simulink model "Modelo_NL_Ley_de_control_NL"  (R2017a)
settings: Solver=VariableStepAuto  StartTime=0.0  StopTime=2  MaxStep=1e-4  RelTol=1e-3
undefined symbols (not defined in the file): alfa_cu, beq, Cts, Jeq, LambdaM, Ld, Lq, Pp, Rs, Rsref, Rts_amb, Tamb, Tleq, Tsref
settings Model: Creator=merem  LastModifiedBy=merem

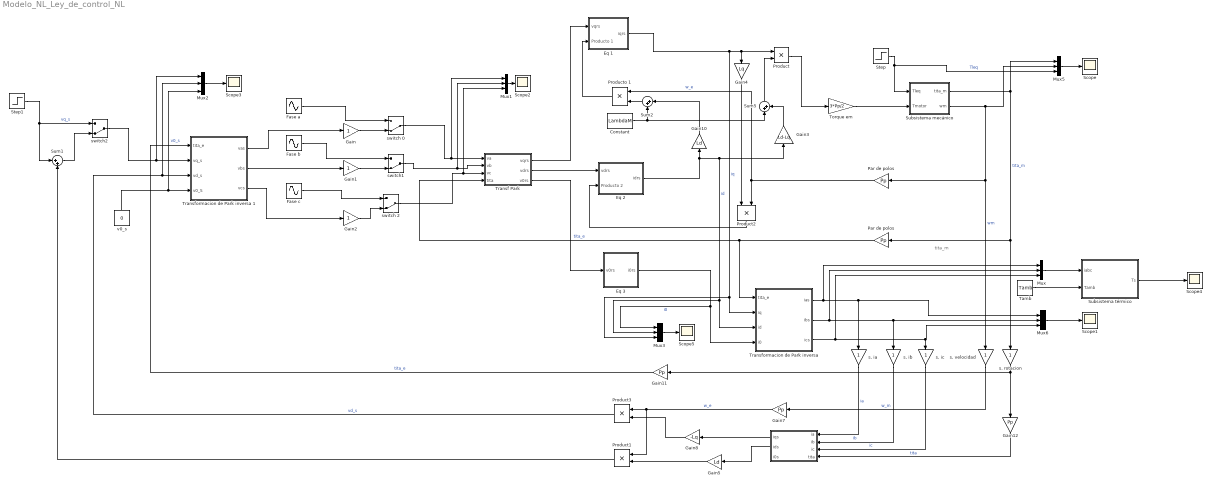
== system Modelo_NL_Ley_de_control_NL ==
  note: tita_m
  " " : Subsystem
  Constant : Constant  Value=LambdaM
  Eq 1 : Subsystem
  "Eq 2 " : Subsystem
  Eq 3 : Subsystem
  Fase a : Sin  SampleTime=0
  Fase b : Sin  SampleTime=0
  Fase c : Sin  SampleTime=0
  Gain : Gain
  Gain1 : Gain
  Gain10 : Gain  Gain=Ld
  Gain11 : Gain  Gain=Pp
  Gain12 : Gain  Gain=Pp
  Gain2 : Gain
  Gain3 : Gain  Gain=Ld-Lq
  Gain4 : Gain  Gain=Lq
  Gain5 : Gain  Gain=Ld
  Gain7 : Gain  Gain=Pp
  Gain8 : Gain  Gain=-Lq
  Mux{,1..3,5..6} (6 alike) : Mux  Inputs=3
  Par de polos : Gain  Gain=Pp
  "Par de polos " : Gain  Gain=Pp
  Product{,1..3} (4 alike) : Product
  Producto 1 : Product
  Scope{,1..5} (6 alike) : Scope
  Step : Step  Time=0  After=Tleq  SampleTime=0
  Step1 : Step  Time=0  After=20  SampleTime=0
  Subsistema mecánico : Subsystem
  Subsistema térmico : Subsystem
  Sum1 : Sum  Inputs=|++
  Sum2 : Sum  Inputs=|++
  Sum5 : Sum  Inputs=|++
  "Tamb " : Constant  Value=Tamb
  "Torque em " : Gain  Gain=3*Pp/2
  "Transf Park " : Subsystem
  "Transformacion de Park inversa " : Subsystem
  Transformacion de Park inversa 1 : Subsystem
  s. ia : Gain
  s. ib : Gain
  "s. ic " : Gain
  s. rotacion : Gain
  s. velocidad : Gain
  switch 0 : ManualSwitch  CurrentSetting=0
  "switch 2 " : ManualSwitch  CurrentSetting=0
  switch1 : ManualSwitch  CurrentSetting=0
  switch2 : ManualSwitch  CurrentSetting=0
  v0_s : Constant  Value=0
  wires:
  s. rotacion/1 -> Gain12/1, Gain11/1
  "s. ic "/1 -> " "/3("ic ")  "ic"
  "Transformacion de Park inversa "/1(ias) -> Mux/1, s. ia/1, Mux6/1
  Sum5/1 -> Product/2
  switch 0/1 -> Mux1/1, "Transf Park "/1("va ")
  Gain7/1 -> Product3/1, Product1/1  "w_e"
  Gain8/1 -> Product3/2
  switch1/1 -> Mux1/2, "Transf Park "/2(vb)
  s. ia/1 -> " "/1("ia ")  "ia"
  s. velocidad/1 -> Gain7/1  "w_m"
  "Torque em "/1 -> Subsistema mecánico/2("Tmotor ")
  Gain5/1 -> Product1/2
  "Eq 2 "/1("idrs ") -> Mux3/2, "Transformacion de Park inversa "/3(id), Gain3/1, Gain10/1  "id"
  Producto 1/1 -> Eq 1/2("Producto 1 ")
  Gain4/1 -> Product2/1
  Subsistema mecánico/1("tita_m ") -> "Par de polos "/1, s. rotacion/1, Mux5/1  "tita_m"
  Gain3/1 -> Sum5/2
  Step/1 -> Mux5/3, Subsistema mecánico/1("Tleq ")  "Tleq"
  Gain10/1 -> Sum2/1
  Eq 1/1("iqrs ") -> Mux3/3, "Transformacion de Park inversa "/2(iq), Gain4/1, Product/1  "iq"
  Gain1/1 -> switch1/2
  Gain2/1 -> "switch 2 "/2
  "switch 2 "/1 -> Mux1/3, "Transf Park "/3(vc)
  Fase c/1 -> "switch 2 "/1
  Product/1 -> "Torque em "/1
  Mux5/1 -> Scope/1
  Gain12/1 -> " "/4("tita ")  "tita"
  "Transformacion de Park inversa "/3("ics ") -> Mux/3, Mux6/3, "s. ic "/1
  v0_s/1 -> Mux2/3, Transformacion de Park inversa 1/4("v0_S ")  "v0_s"
  Product3/1 -> Mux2/2, Transformacion de Park inversa 1/3(vd_s)  "vd_s"
  s. ib/1 -> " "/2("ib ")  "ib"
  Fase b/1 -> switch1/1
  Par de polos/1 -> Producto 1/1, Product2/2  "w_e"
  Constant/1 -> Sum5/1, Sum2/2
  Mux6/1 -> Scope1/1
  Gain11/1 -> Transformacion de Park inversa 1/1(tita_e)  "tita_e"
  "Transf Park "/2("vdrs ") -> "Eq 2 "/1("vdrs ")
  Gain/1 -> switch 0/2
  Fase a/1 -> switch 0/1
  " "/2("ids ") -> Gain5/1
  "Transf Park "/1(vqrs) -> Eq 1/1(vqrs)
  "Par de polos "/1 -> "Transf Park "/4(tita), "Transformacion de Park inversa "/1(tita_e)  "tita_e"
  Transformacion de Park inversa 1/1(vas) -> Gain/1
  Mux/1 -> Subsistema térmico/1(iabc)
  Transformacion de Park inversa 1/3("vcs ") -> Gain2/1
  " "/1(iqs) -> Gain8/1
  Subsistema térmico/1(Ts) -> Scope4/1
  Eq 3/1("i0rs ") -> Mux3/1, "Transformacion de Park inversa "/4(i0)  "i0"
  Product2/1 -> "Eq 2 "/2("Producto 2 ")
  "Transformacion de Park inversa "/2(ibs) -> Mux/2, Mux6/2, s. ib/1
  Mux1/1 -> Scope2/1
  Sum2/1 -> Producto 1/2
  "Transf Park "/3("v0rs ") -> Eq 3/1("v0rs ")
  Mux2/1 -> Scope3/1
  Transformacion de Park inversa 1/2(vbs) -> Gain1/1
  Subsistema mecánico/2("wm ") -> Par de polos/1, s. velocidad/1, Mux5/2  "wm"
  Product1/1 -> Sum1/2
  "Tamb "/1 -> Subsistema térmico/2("Tamb ")
  Mux3/1 -> Scope5/1
  Step1/1 -> switch2/1, Sum1/1  "vq_s"
  switch2/1 -> Mux2/1, Transformacion de Park inversa 1/2(vq_s)
  Sum1/1 -> switch2/2

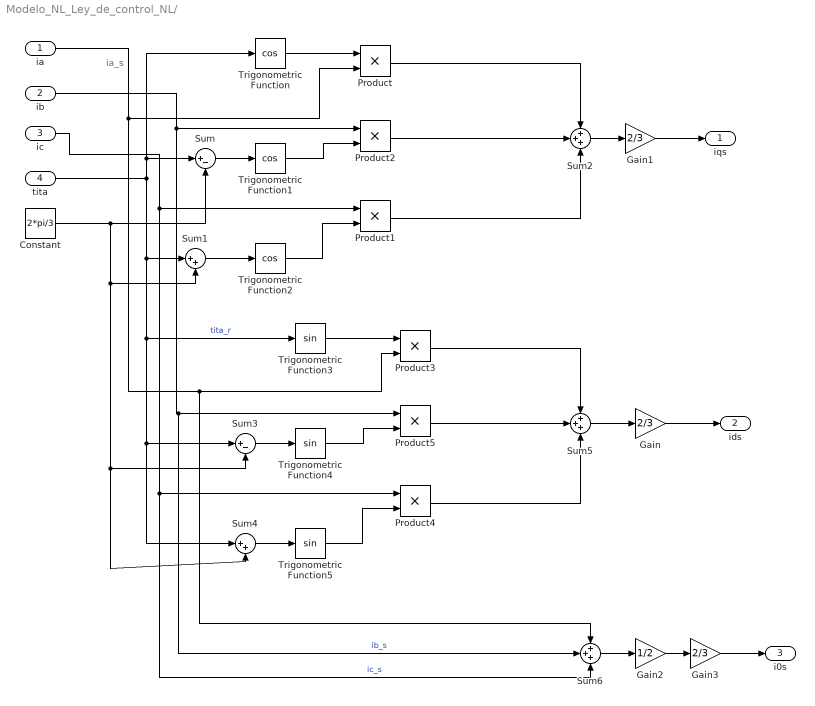
== system Modelo_NL_Ley_de_control_NL/  ==
  note: ia_s
  "ia " : Inport
  "ib " : Inport  Port=2
  "ic " : Inport  Port=3
  "tita " : Inport  Port=4
  Constant : Constant  Value=2*pi/3
  Gain : Gain  Gain=2/3
  Gain1 : Gain  Gain=2/3
  Gain2 : Gain  Gain=1/2
  Gain3 : Gain  Gain=2/3
  Product{,1..5} (6 alike) : Product
  Sum : Sum  Inputs=|+-
  Sum1 : Sum  Inputs=|++
  Sum2 : Sum  Inputs=+++
  Sum3 : Sum  Inputs=|+-
  Sum4 : Sum  Inputs=|++
  Sum5 : Sum  Inputs=+++
  Sum6 : Sum  Inputs=+++
  Trigonometric Function : Trigonometry  Operator=cos
  Trigonometric Function1 : Trigonometry  Operator=cos
  Trigonometric Function2 : Trigonometry  Operator=cos
  Trigonometric Function3 : Trigonometry
  Trigonometric Function4 : Trigonometry
  Trigonometric Function5 : Trigonometry
  iqs : Outport
  "ids " : Outport  Port=2
  "i0s " : Outport  Port=3
  wires:
  "tita "/1 -> Trigonometric Function/1, Sum/1, Sum1/1, Trigonometric Function3/1, Sum3/1, Sum4/1  "tita_r"
  Trigonometric Function/1 -> Product/1
  "ia "/1 -> Sum6/1, Product3/2, Product/2
  Constant/1 -> Sum4/2, Sum3/2, Sum1/2, Sum/2
  Sum/1 -> Trigonometric Function1/1
  Sum1/1 -> Trigonometric Function2/1
  Trigonometric Function1/1 -> Product2/2
  Trigonometric Function2/1 -> Product1/2
  "ib "/1 -> Sum6/2, Product5/1, Product2/1  "ib_s"
  "ic "/1 -> Sum6/3, Product4/1, Product1/1  "ic_s"
  Product/1 -> Sum2/1
  Product2/1 -> Sum2/2
  Sum2/1 -> Gain1/1
  Trigonometric Function5/1 -> Product4/2
  Trigonometric Function3/1 -> Product3/1
  Sum4/1 -> Trigonometric Function5/1
  Sum3/1 -> Trigonometric Function4/1
  Trigonometric Function4/1 -> Product5/2
  Product3/1 -> Sum5/1
  Product5/1 -> Sum5/2
  Product4/1 -> Sum5/3
  Sum5/1 -> Gain/1
  Product1/1 -> Sum2/3
  Gain/1 -> "ids "/1
  Gain1/1 -> iqs/1
  Sum6/1 -> Gain2/1
  Gain2/1 -> Gain3/1
  Gain3/1 -> "i0s "/1

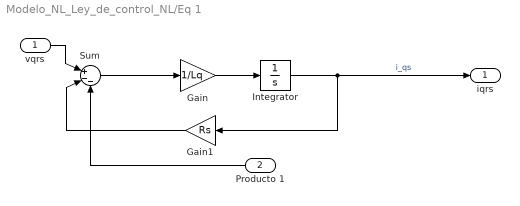
== system Modelo_NL_Ley_de_control_NL/Eq 1 ==
  vqrs : Inport
  "Producto 1 " : Inport  Port=2
  Gain : Gain  Gain=1/Lq
  Gain1 : Gain  Gain=Rs
  Integrator : Integrator
  Sum : Sum  Inputs=|+--
  "iqrs " : Outport
  wires:
  Gain/1 -> Integrator/1
  Sum/1 -> Gain/1
  vqrs/1 -> Sum/1
  Gain1/1 -> Sum/2
  "Producto 1 "/1 -> Sum/3
  Integrator/1 -> "iqrs "/1, Gain1/1  "i_qs"

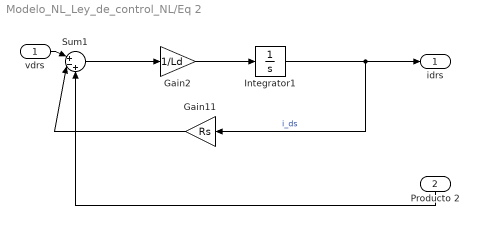
== system Modelo_NL_Ley_de_control_NL/Eq 2  ==
  "vdrs " : Inport
  "Producto 2 " : Inport  Port=2
  Gain11 : Gain  Gain=Rs
  Gain2 : Gain  Gain=1/Ld
  Integrator1 : Integrator
  Sum1 : Sum  Inputs=|+-+
  "idrs " : Outport
  wires:
  "Producto 2 "/1 -> Sum1/3
  Gain2/1 -> Integrator1/1
  Gain11/1 -> Sum1/2
  Sum1/1 -> Gain2/1
  Integrator1/1 -> Gain11/1, "idrs "/1  "i_ds"
  "vdrs "/1 -> Sum1/1

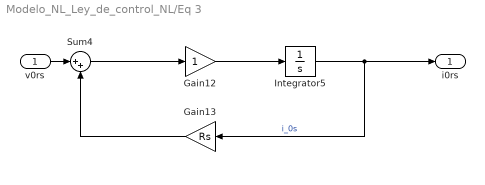
== system Modelo_NL_Ley_de_control_NL/Eq 3 ==
  "v0rs " : Inport
  Gain12 : Gain
  Gain13 : Gain  Gain=Rs
  Integrator5 : Integrator
  Sum4 : Sum  Inputs=|++
  "i0rs " : Outport
  wires:
  Gain12/1 -> Integrator5/1
  Sum4/1 -> Gain12/1
  Gain13/1 -> Sum4/2
  "v0rs "/1 -> Sum4/1
  Integrator5/1 -> "i0rs "/1, Gain13/1  "i_0s"

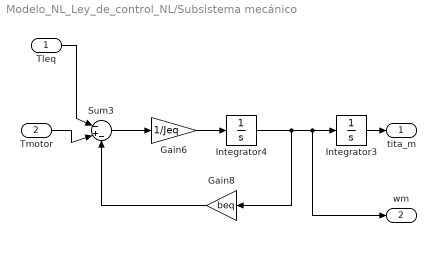
== system Modelo_NL_Ley_de_control_NL/Subsistema mecánico ==
  "Tleq " : Inport
  "Tmotor " : Inport  Port=2
  Gain6 : Gain  Gain=1/Jeq
  Gain8 : Gain  Gain=beq
  Integrator3 : Integrator
  Integrator4 : Integrator
  Sum3 : Sum  Inputs=|-+-
  "tita_m " : Outport
  "wm " : Outport  Port=2
  wires:
  Integrator3/1 -> "tita_m "/1
  Integrator4/1 -> Gain8/1, "wm "/1, Integrator3/1
  Sum3/1 -> Gain6/1
  Gain6/1 -> Integrator4/1
  Gain8/1 -> Sum3/3
  "Tleq "/1 -> Sum3/1
  "Tmotor "/1 -> Sum3/2

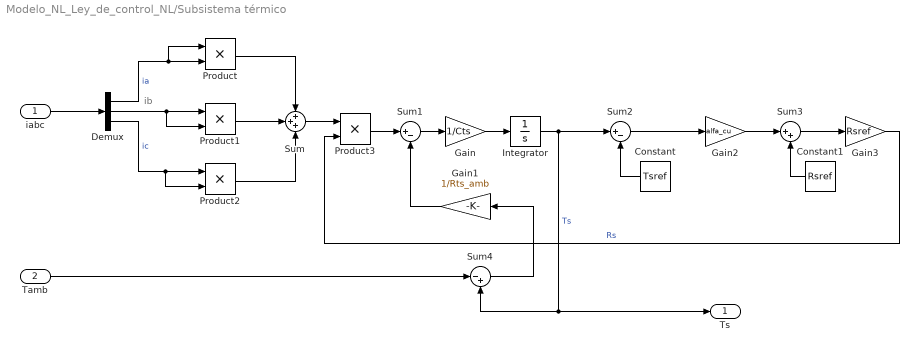
== system Modelo_NL_Ley_de_control_NL/Subsistema térmico ==
  note: ib
  iabc : Inport
  "Tamb " : Inport  Port=2
  Constant : Constant  Value=Tsref
  Constant1 : Constant  Value=Rsref
  Demux : Demux  Outputs=3
  Gain : Gain  Gain=1/Cts
  Gain1 : Gain  Gain=1/Rts_amb
  Gain2 : Gain  Gain=alfa_cu
  Gain3 : Gain  Gain=Rsref
  Integrator : Integrator
  Product{,1..3} (4 alike) : Product
  Sum : Sum  Inputs=+++
  Sum1 : Sum  Inputs=|+-
  Sum2 : Sum  Inputs=|+-
  Sum3 : Sum  Inputs=|++
  Sum4 : Sum  Inputs=|-+
  Ts : Outport
  wires:
  iabc/1 -> Demux/1
  Demux/1 -> Product/2, Product/1  "ia"
  Demux/2 -> Product1/2, Product1/1
  Demux/3 -> Product2/2, Product2/1  "ic"
  Product/1 -> Sum/1
  Product1/1 -> Sum/2
  Product2/1 -> Sum/3
  Sum/1 -> Product3/1
  Gain/1 -> Integrator/1
  Product3/1 -> Sum1/1
  Sum1/1 -> Gain/1
  Gain1/1 -> Sum1/2
  Integrator/1 -> Ts/1, Sum4/2, Sum2/1  "Ts"
  Constant/1 -> Sum2/2
  Sum2/1 -> Gain2/1
  Gain2/1 -> Sum3/1
  Constant1/1 -> Sum3/2
  Sum3/1 -> Gain3/1
  Gain3/1 -> Product3/2  "Rs"
  "Tamb "/1 -> Sum4/1
  Sum4/1 -> Gain1/1

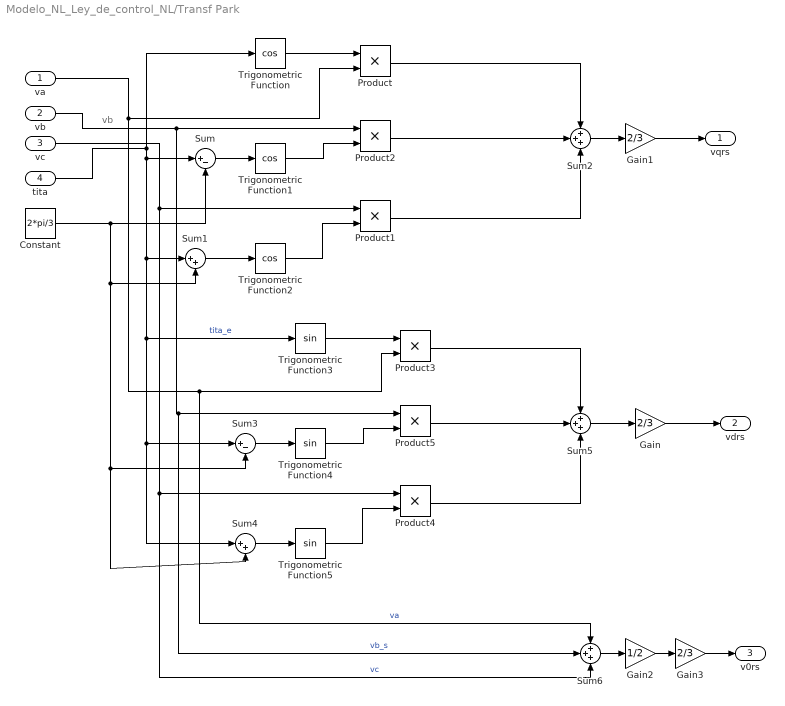
== system Modelo_NL_Ley_de_control_NL/Transf Park  ==
  note: vb
  "va " : Inport
  vb : Inport  Port=2
  vc : Inport  Port=3
  tita : Inport  Port=4
  Constant : Constant  Value=2*pi/3
  Gain : Gain  Gain=2/3
  Gain1 : Gain  Gain=2/3
  Gain2 : Gain  Gain=1/2
  Gain3 : Gain  Gain=2/3
  Product{,1..5} (6 alike) : Product
  Sum : Sum  Inputs=|+-
  Sum1 : Sum  Inputs=|++
  Sum2 : Sum  Inputs=+++
  Sum3 : Sum  Inputs=|+-
  Sum4 : Sum  Inputs=|++
  Sum5 : Sum  Inputs=+++
  Sum6 : Sum  Inputs=+++
  Trigonometric Function : Trigonometry  Operator=cos
  Trigonometric Function1 : Trigonometry  Operator=cos
  Trigonometric Function2 : Trigonometry  Operator=cos
  Trigonometric Function3 : Trigonometry
  Trigonometric Function4 : Trigonometry
  Trigonometric Function5 : Trigonometry
  vqrs : Outport
  "vdrs " : Outport  Port=2
  "v0rs " : Outport  Port=3
  wires:
  tita/1 -> Sum1/1, Trigonometric Function3/1, Sum3/1, Sum4/1, Sum/1, Trigonometric Function/1  "tita_e"
  Trigonometric Function/1 -> Product/1
  "va "/1 -> Sum6/1, Product3/2, Product/2  "va"
  Constant/1 -> Sum4/2, Sum3/2, Sum1/2, Sum/2
  Sum/1 -> Trigonometric Function1/1
  Sum1/1 -> Trigonometric Function2/1
  Trigonometric Function1/1 -> Product2/2
  Trigonometric Function2/1 -> Product1/2
  vb/1 -> Sum6/2, Product5/1, Product2/1  "vb_s"
  vc/1 -> Sum6/3, Product4/1, Product1/1  "vc"
  Product/1 -> Sum2/1
  Product2/1 -> Sum2/2
  Sum2/1 -> Gain1/1
  Trigonometric Function5/1 -> Product4/2
  Trigonometric Function3/1 -> Product3/1
  Sum4/1 -> Trigonometric Function5/1
  Sum3/1 -> Trigonometric Function4/1
  Trigonometric Function4/1 -> Product5/2
  Product3/1 -> Sum5/1
  Product5/1 -> Sum5/2
  Product4/1 -> Sum5/3
  Sum5/1 -> Gain/1
  Product1/1 -> Sum2/3
  Gain/1 -> "vdrs "/1
  Gain1/1 -> vqrs/1
  Sum6/1 -> Gain2/1
  Gain3/1 -> "v0rs "/1
  Gain2/1 -> Gain3/1

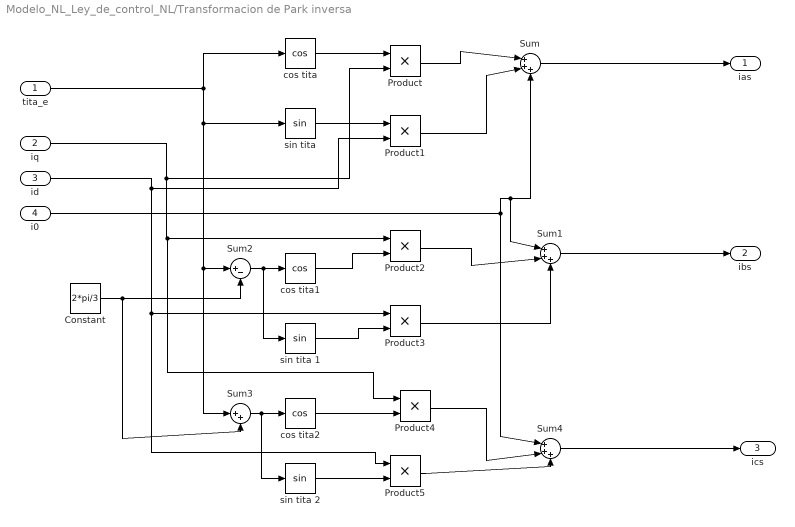
== system Modelo_NL_Ley_de_control_NL/Transformacion de Park inversa  ==
  tita_e : Inport
  iq : Inport  Port=2
  id : Inport  Port=3
  i0 : Inport  Port=4
  Constant : Constant  Value=2*pi/3
  Product{,1..5} (6 alike) : Product
  Sum : Sum  Inputs=|+++
  Sum1 : Sum  Inputs=|+++
  Sum2 : Sum  Inputs=|+-
  Sum3 : Sum  Inputs=|++
  Sum4 : Sum  Inputs=|+++
  cos tita : Trigonometry  Operator=cos
  cos tita1 : Trigonometry  Operator=cos
  cos tita2 : Trigonometry  Operator=cos
  "sin tita " : Trigonometry
  sin tita 1 : Trigonometry
  sin tita 2 : Trigonometry
  ias : Outport
  ibs : Outport  Port=2
  "ics " : Outport  Port=3
  wires:
  tita_e/1 -> Sum3/1, Sum2/1, "sin tita "/1, cos tita/1
  iq/1 -> Product4/1, Product2/1, Product/2
  cos tita/1 -> Product/1
  "sin tita "/1 -> Product1/1
  id/1 -> Product5/1, Product3/1, Product1/2
  Product/1 -> Sum/1
  Product1/1 -> Sum/2
  Sum/1 -> ias/1
  i0/1 -> Sum1/1, Sum/3, Sum4/1
  cos tita1/1 -> Product2/2
  sin tita 1/1 -> Product3/2
  Product3/1 -> Sum1/3
  Product2/1 -> Sum1/2
  Sum1/1 -> ibs/1
  Constant/1 -> Sum3/2, Sum2/2
  Sum2/1 -> sin tita 1/1, cos tita1/1
  Sum3/1 -> sin tita 2/1, cos tita2/1
  cos tita2/1 -> Product4/2
  sin tita 2/1 -> Product5/2
  Product5/1 -> Sum4/3
  Product4/1 -> Sum4/2
  Sum4/1 -> "ics "/1

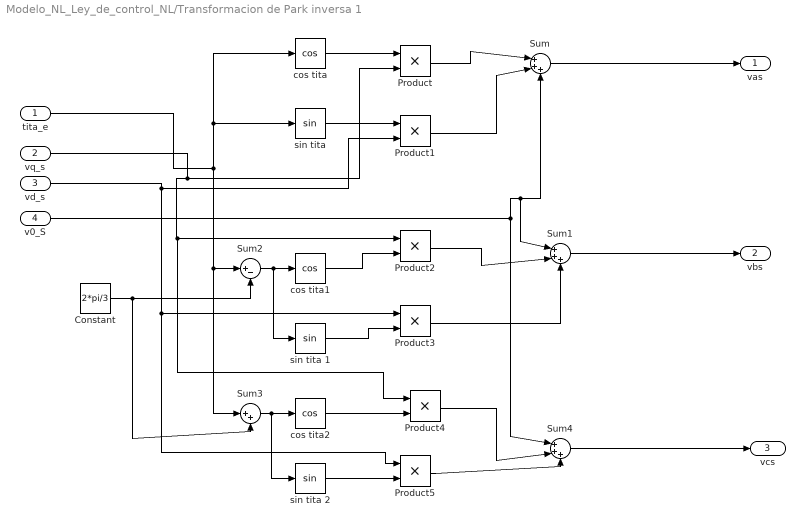
== system Modelo_NL_Ley_de_control_NL/Transformacion de Park inversa 1 ==
  tita_e : Inport
  vq_s : Inport  Port=2
  vd_s : Inport  Port=3
  "v0_S " : Inport  Port=4
  Constant : Constant  Value=2*pi/3
  Product{,1..5} (6 alike) : Product
  Sum : Sum  Inputs=|+++
  Sum1 : Sum  Inputs=|+++
  Sum2 : Sum  Inputs=|+-
  Sum3 : Sum  Inputs=|++
  Sum4 : Sum  Inputs=|+++
  cos tita : Trigonometry  Operator=cos
  cos tita1 : Trigonometry  Operator=cos
  cos tita2 : Trigonometry  Operator=cos
  "sin tita " : Trigonometry
  sin tita 1 : Trigonometry
  sin tita 2 : Trigonometry
  vas : Outport
  vbs : Outport  Port=2
  "vcs " : Outport  Port=3
  wires:
  tita_e/1 -> Sum3/1, Sum2/1, cos tita/1, "sin tita "/1
  vq_s/1 -> Product4/1, Product2/1, Product/2
  cos tita/1 -> Product/1
  "sin tita "/1 -> Product1/1
  vd_s/1 -> Product5/1, Product3/1, Product1/2
  Product/1 -> Sum/1
  Product1/1 -> Sum/2
  Sum/1 -> vas/1
  "v0_S "/1 -> Sum1/1, Sum/3, Sum4/1
  cos tita1/1 -> Product2/2
  sin tita 1/1 -> Product3/2
  Product3/1 -> Sum1/3
  Product2/1 -> Sum1/2
  Sum1/1 -> vbs/1
  Constant/1 -> Sum3/2, Sum2/2
  Sum2/1 -> sin tita 1/1, cos tita1/1
  Sum3/1 -> sin tita 2/1, cos tita2/1
  cos tita2/1 -> Product4/2
  sin tita 2/1 -> Product5/2
  Product5/1 -> Sum4/3
  Product4/1 -> Sum4/2
  Sum4/1 -> "vcs "/1
